simulink model "Gate_Splitter_x4"  (Simulink 6.6)
settings: Solver=ode45  StartTime=0.0  StopTime=5000/144e6  RelTol=1e-3
libraries: xbsIndex_r4 x205, simulink x1
(part 1 of 2)
settings Model: Creator=tbrimeye  LastModifiedBy=tbrimeye
settings DebuggingCC: SignalResolutionControl=TryResolveAllWithWarning  MultiTaskDSMMsg=warning  MultiTaskCondExecSysMsg=none
settings RTWCC: IncludeERTFirstTime=on

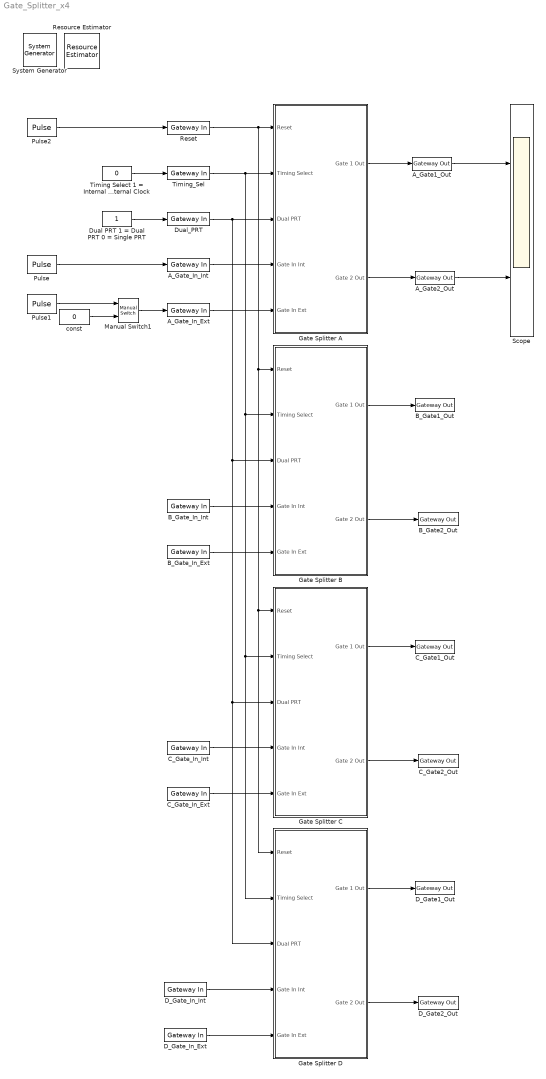
== system Gate_Splitter_x4 ==
  " System Generator" : xbsIndex_r4/ System Generator  Tag=genX  SystemSampleTime=-1  xilinxfamily=virtex4  part=xc4vsx35  speed=-11  package=ff668  synthesis_tool=XST  directory=C:/Work_Projects/Xilinx/SysGen_Outputs/Gate_Splitter  testbench=off  simulink_period=1/60e6  sysclk_period=(1/60e6)*1e9  incr_netlist=off  trim_vbits=Everywhere in SubSystem  dbl_ovrd=According to Block Masks  core_generation=According to Block Masks  run_coregen=off  deprecated_control=off  eval_field=0  block_type=sysgen
      settings: block_version=8.2
  A_Gate1_Out : xbsIndex_r4/Gateway Out  hdl_port=on  timing_constraint=None  locs_specified=off  LOCs={}  block_type=gatewayout
      settings: infoedit="Gateway out block.  Converts Xilinx fixed point inputs into ouputs of type Simulink integer, double, or fixed point.<P><P>Hardware notes:  In hardware these blocks become top level output ports or are discarded, depending on how they are configured."  xl_area=[0 0 0 0 18 0 0]  block_version=VER_STRING_GOES_HERE
  A_Gate2_Out : xbsIndex_r4/Gateway Out  hdl_port=on  timing_constraint=None  locs_specified=off  LOCs={}  block_type=gatewayout
      settings: infoedit="Gateway out block.  Converts Xilinx fixed point inputs into ouputs of type Simulink integer, double, or fixed point.<P><P>Hardware notes:  In hardware these blocks become top level output ports or are discarded, depending on how they are configured."  xl_area=[0 0 0 0 18 0 0]  block_version=VER_STRING_GOES_HERE
  A_Gate_In_Ext : xbsIndex_r4/Gateway In  arith_type=Boolean  n_bits=18  bin_pt=0  quantization="Round  (unbiased: +/- Inf)"  overflow=Flag as error  period=1/60e6  dbl_ovrd=off  timing_constraint=None  locs_specified=off  LOCs={}  block_type=gatewayin
      settings: infoedit="Gateway in block.  Converts inputs of type Simulink integer, double and fixed point to  Xilinx fixed point type.<P><P>Hardware notes:  In hardware these blocks become top level input ports."  xl_area=[0 0 0 0 1 0 0]  block_version=8.2
  A_Gate_In_Int : xbsIndex_r4/Gateway In  arith_type=Boolean  n_bits=1  bin_pt=0  quantization="Round  (unbiased: +/- Inf)"  overflow=Flag as error  period=1/60e6  dbl_ovrd=off  timing_constraint=None  locs_specified=off  LOCs={}  block_type=gatewayin
      settings: infoedit="Gateway in block.  Converts inputs of type Simulink integer, double and fixed point to  Xilinx fixed point type.<P><P>Hardware notes:  In hardware these blocks become top level input ports."  xl_area=[0 0 0 0 1 0 0]  block_version=8.2
  B_Gate1_Out : xbsIndex_r4/Gateway Out  hdl_port=on  timing_constraint=None  locs_specified=off  LOCs={}  block_type=gatewayout
      settings: infoedit="Gateway out block.  Converts Xilinx fixed point inputs into ouputs of type Simulink integer, double, or fixed point.<P><P>Hardware notes:  In hardware these blocks become top level output ports or are discarded, depending on how they are configured."  xl_area=[0 0 0 0 18 0 0]  block_version=VER_STRING_GOES_HERE
  B_Gate2_Out : xbsIndex_r4/Gateway Out  hdl_port=on  timing_constraint=None  locs_specified=off  LOCs={}  block_type=gatewayout
      settings: infoedit="Gateway out block.  Converts Xilinx fixed point inputs into ouputs of type Simulink integer, double, or fixed point.<P><P>Hardware notes:  In hardware these blocks become top level output ports or are discarded, depending on how they are configured."  xl_area=[0 0 0 0 18 0 0]  block_version=VER_STRING_GOES_HERE
  B_Gate_In_Ext : xbsIndex_r4/Gateway In  arith_type=Boolean  n_bits=18  bin_pt=0  quantization="Round  (unbiased: +/- Inf)"  overflow=Flag as error  period=1/60e6  dbl_ovrd=off  timing_constraint=None  locs_specified=off  LOCs={}  block_type=gatewayin
      settings: infoedit="Gateway in block.  Converts inputs of type Simulink integer, double and fixed point to  Xilinx fixed point type.<P><P>Hardware notes:  In hardware these blocks become top level input ports."  xl_area=[0 0 0 0 1 0 0]  block_version=8.2
  B_Gate_In_Int : xbsIndex_r4/Gateway In  arith_type=Boolean  n_bits=1  bin_pt=0  quantization="Round  (unbiased: +/- Inf)"  overflow=Flag as error  period=1/60e6  dbl_ovrd=off  timing_constraint=None  locs_specified=off  LOCs={}  block_type=gatewayin
      settings: infoedit="Gateway in block.  Converts inputs of type Simulink integer, double and fixed point to  Xilinx fixed point type.<P><P>Hardware notes:  In hardware these blocks become top level input ports."  xl_area=[0 0 0 0 1 0 0]  block_version=8.2
  C_Gate1_Out : xbsIndex_r4/Gateway Out  hdl_port=on  timing_constraint=None  locs_specified=off  LOCs={}  block_type=gatewayout
      settings: infoedit="Gateway out block.  Converts Xilinx fixed point inputs into ouputs of type Simulink integer, double, or fixed point.<P><P>Hardware notes:  In hardware these blocks become top level output ports or are discarded, depending on how they are configured."  xl_area=[0 0 0 0 18 0 0]  block_version=VER_STRING_GOES_HERE
  C_Gate2_Out : xbsIndex_r4/Gateway Out  hdl_port=on  timing_constraint=None  locs_specified=off  LOCs={}  block_type=gatewayout
      settings: infoedit="Gateway out block.  Converts Xilinx fixed point inputs into ouputs of type Simulink integer, double, or fixed point.<P><P>Hardware notes:  In hardware these blocks become top level output ports or are discarded, depending on how they are configured."  xl_area=[0 0 0 0 18 0 0]  block_version=VER_STRING_GOES_HERE
  C_Gate_In_Ext : xbsIndex_r4/Gateway In  arith_type=Boolean  n_bits=18  bin_pt=0  quantization="Round  (unbiased: +/- Inf)"  overflow=Flag as error  period=1/60e6  dbl_ovrd=off  timing_constraint=None  locs_specified=off  LOCs={}  block_type=gatewayin
      settings: infoedit="Gateway in block.  Converts inputs of type Simulink integer, double and fixed point to  Xilinx fixed point type.<P><P>Hardware notes:  In hardware these blocks become top level input ports."  xl_area=[0 0 0 0 1 0 0]  block_version=8.2
  C_Gate_In_Int : xbsIndex_r4/Gateway In  arith_type=Boolean  n_bits=1  bin_pt=0  quantization="Round  (unbiased: +/- Inf)"  overflow=Flag as error  period=1/60e6  dbl_ovrd=off  timing_constraint=None  locs_specified=off  LOCs={}  block_type=gatewayin
      settings: infoedit="Gateway in block.  Converts inputs of type Simulink integer, double and fixed point to  Xilinx fixed point type.<P><P>Hardware notes:  In hardware these blocks become top level input ports."  xl_area=[0 0 0 0 1 0 0]  block_version=8.2
  D_Gate1_Out : xbsIndex_r4/Gateway Out  hdl_port=on  timing_constraint=None  locs_specified=off  LOCs={}  block_type=gatewayout
      settings: infoedit="Gateway out block.  Converts Xilinx fixed point inputs into ouputs of type Simulink integer, double, or fixed point.<P><P>Hardware notes:  In hardware these blocks become top level output ports or are discarded, depending on how they are configured."  xl_area=[0 0 0 0 18 0 0]  block_version=VER_STRING_GOES_HERE
  D_Gate2_Out : xbsIndex_r4/Gateway Out  hdl_port=on  timing_constraint=None  locs_specified=off  LOCs={}  block_type=gatewayout
      settings: infoedit="Gateway out block.  Converts Xilinx fixed point inputs into ouputs of type Simulink integer, double, or fixed point.<P><P>Hardware notes:  In hardware these blocks become top level output ports or are discarded, depending on how they are configured."  xl_area=[0 0 0 0 18 0 0]  block_version=VER_STRING_GOES_HERE
  D_Gate_In_Ext : xbsIndex_r4/Gateway In  arith_type=Boolean  n_bits=18  bin_pt=0  quantization="Round  (unbiased: +/- Inf)"  overflow=Flag as error  period=1/60e6  dbl_ovrd=off  timing_constraint=None  locs_specified=off  LOCs={}  block_type=gatewayin
      settings: infoedit="Gateway in block.  Converts inputs of type Simulink integer, double and fixed point to  Xilinx fixed point type.<P><P>Hardware notes:  In hardware these blocks become top level input ports."  xl_area=[0 0 0 0 1 0 0]  block_version=8.2
  D_Gate_In_Int : xbsIndex_r4/Gateway In  arith_type=Boolean  n_bits=1  bin_pt=0  quantization="Round  (unbiased: +/- Inf)"  overflow=Flag as error  period=1/60e6  dbl_ovrd=off  timing_constraint=None  locs_specified=off  LOCs={}  block_type=gatewayin
      settings: infoedit="Gateway in block.  Converts inputs of type Simulink integer, double and fixed point to  Xilinx fixed point type.<P><P>Hardware notes:  In hardware these blocks become top level input ports."  xl_area=[0 0 0 0 1 0 0]  block_version=8.2
  Dual PRT 1 = Dual PRT 0 = Single PRT : Constant
  Dual_PRT : xbsIndex_r4/Gateway In  arith_type=Boolean  n_bits=1  bin_pt=0  quantization="Round  (unbiased: +/- Inf)"  overflow=Flag as error  period=1/60e6  dbl_ovrd=off  timing_constraint=None  locs_specified=off  LOCs={}  block_type=gatewayin
      settings: infoedit="Gateway in block.  Converts inputs of type Simulink integer, double and fixed point to  Xilinx fixed point type.<P><P>Hardware notes:  In hardware these blocks become top level input ports."  xl_area=[0 0 0 0 1 0 0]  block_version=8.2
  Gate Splitter A : Subsystem
  Gate Splitter B : Subsystem
  Gate Splitter C : Subsystem
  Gate Splitter D : Subsystem
  Manual Switch1 : simulink/Signal Routing/Manual Switch  SystemSampleTime=-1  sw=1  action=0  varsize=off
  Pulse : DiscretePulseGenerator  PulseType=Time based  Period=500/144e6  PulseWidth=50  PhaseDelay=100/144e6
  Pulse1 : DiscretePulseGenerator  PulseType=Time based  Period=500/144e6  PulseWidth=20  PhaseDelay=100/144e6
  Pulse2 : DiscretePulseGenerator  PulseType=Time based  Period=5000/144e6
  Reset : xbsIndex_r4/Gateway In  arith_type=Boolean  n_bits=1  bin_pt=0  quantization="Round  (unbiased: +/- Inf)"  overflow=Flag as error  period=1/60e6  dbl_ovrd=off  timing_constraint=None  locs_specified=off  LOCs={}  block_type=gatewayin
      settings: infoedit="Gateway in block.  Converts inputs of type Simulink integer, double and fixed point to  Xilinx fixed point type.<P><P>Hardware notes:  In hardware these blocks become top level input ports."  xl_area=[0 0 0 0 1 0 0]  block_version=8.2
  Resource Estimator : xbsIndex_r4/Resource Estimator  Tag=resEstTag  Slices=925  FFs=1405  BRAMs=7  LUTs=1104  IOBs=133  EBMs=14  TBUFs=0  xl_use_estimator_area=off  est_options=Post Map  xl_estimator_area=[1915 2342 0 3405 33 4 0]  block_type=resource_estimator
      settings: AttributesFormatString=Resource\nEstimator  block_version=8.2
  Scope : Scope  NumInputPorts=2
      settings: YMin=-5~-5  YMax=5~5
  Timing Select 1 = Internal Clock 0 = External Clock : Constant  Value=0
  Timing_Sel : xbsIndex_r4/Gateway In  arith_type=Boolean  n_bits=1  bin_pt=0  quantization="Round  (unbiased: +/- Inf)"  overflow=Flag as error  period=1/60e6  dbl_ovrd=off  timing_constraint=None  locs_specified=off  LOCs={}  block_type=gatewayin
      settings: infoedit="Gateway in block.  Converts inputs of type Simulink integer, double and fixed point to  Xilinx fixed point type.<P><P>Hardware notes:  In hardware these blocks become top level input ports."  xl_area=[0 0 0 0 1 0 0]  block_version=8.2
  const : Constant  Value=0
  wires:
  Pulse/1 -> A_Gate_In_Int/1
  Pulse1/1 -> Manual Switch1/1
  const/1 -> Manual Switch1/2
  Manual Switch1/1 -> A_Gate_In_Ext/1
  Dual PRT 1 = Dual PRT 0 = Single PRT/1 -> Dual_PRT/1
  Timing Select 1 = Internal Clock 0 = External Clock/1 -> Timing_Sel/1
  Pulse2/1 -> Reset/1
  Reset/1 -> Gate Splitter C/1(Reset), Gate Splitter D/1(Reset), Gate Splitter B/1(Reset), Gate Splitter A/1(Reset)
  Timing_Sel/1 -> Gate Splitter C/2(Timing Select), Gate Splitter D/2(Timing Select), Gate Splitter B/2(Timing Select), Gate Splitter A/2(Timing Select)
  Dual_PRT/1 -> Gate Splitter C/3(Dual PRT), Gate Splitter D/3(Dual PRT), Gate Splitter B/3(Dual PRT), Gate Splitter A/3(Dual PRT)
  A_Gate_In_Int/1 -> Gate Splitter A/4(Gate In Int)
  A_Gate_In_Ext/1 -> Gate Splitter A/5(Gate In Ext)
  Gate Splitter A/1(Gate 1 Out) -> A_Gate1_Out/1
  Gate Splitter A/2(Gate 2 Out) -> A_Gate2_Out/1
  B_Gate_In_Int/1 -> Gate Splitter B/4(Gate In Int)
  B_Gate_In_Ext/1 -> Gate Splitter B/5(Gate In Ext)
  C_Gate_In_Int/1 -> Gate Splitter C/4(Gate In Int)
  C_Gate_In_Ext/1 -> Gate Splitter C/5(Gate In Ext)
  D_Gate_In_Int/1 -> Gate Splitter D/4(Gate In Int)
  D_Gate_In_Ext/1 -> Gate Splitter D/5(Gate In Ext)
  Gate Splitter B/1(Gate 1 Out) -> B_Gate1_Out/1
  Gate Splitter B/2(Gate 2 Out) -> B_Gate2_Out/1
  Gate Splitter C/1(Gate 1 Out) -> C_Gate1_Out/1
  Gate Splitter C/2(Gate 2 Out) -> C_Gate2_Out/1
  Gate Splitter D/1(Gate 1 Out) -> D_Gate1_Out/1
  Gate Splitter D/2(Gate 2 Out) -> D_Gate2_Out/1
  A_Gate1_Out/1 -> Scope/1
  A_Gate2_Out/1 -> Scope/2

== system Gate_Splitter_x4/Gate Splitter A ==
  Reset : Inport
  Timing Select : Inport  Port=2
  Dual PRT : Inport  Port=3
  Gate In Int : Inport  Port=4
  Gate In Ext : Inport  Port=5
  Gate Splitter : Subsystem
  Noise Cancellation : Subsystem
  Noise Cancellation1 : Subsystem
  Gate 1 Out : Outport
  Gate 2 Out : Outport  Port=2
  wires:
  Noise Cancellation/1(Gate Out) -> Gate Splitter/4(Gate In Int)
  Noise Cancellation1/1(Gate Out) -> Gate Splitter/5(Gate In Ext)
  Reset/1 -> Gate Splitter/1(Reset)
  Gate In Int/1 -> Noise Cancellation/1(Gate In)
  Gate In Ext/1 -> Noise Cancellation1/1(Gate In)
  Gate Splitter/1(Gate 1 Out) -> Gate 1 Out/1
  Timing Select/1 -> Gate Splitter/2(Timing Sel)
  Dual PRT/1 -> Gate Splitter/3(Dual PRT)
  Gate Splitter/2(Gate 2 Out) -> Gate 2 Out/1

== system Gate_Splitter_x4/Gate Splitter B ==
  Reset : Inport
  Timing Select : Inport  Port=2
  Dual PRT : Inport  Port=3
  Gate In Int : Inport  Port=4
  Gate In Ext : Inport  Port=5
  Gate Splitter : Subsystem
  Noise Cancellation : Subsystem
  Noise Cancellation1 : Subsystem
  Gate 1 Out : Outport
  Gate 2 Out : Outport  Port=2
  wires:
  Noise Cancellation/1(Gate Out) -> Gate Splitter/4(Gate In Int)
  Noise Cancellation1/1(Gate Out) -> Gate Splitter/5(Gate In Ext)
  Reset/1 -> Gate Splitter/1(Reset)
  Gate In Int/1 -> Noise Cancellation/1(Gate In)
  Gate In Ext/1 -> Noise Cancellation1/1(Gate In)
  Gate Splitter/1(Gate 1 Out) -> Gate 1 Out/1
  Timing Select/1 -> Gate Splitter/2(Timing Sel)
  Dual PRT/1 -> Gate Splitter/3(Dual PRT)
  Gate Splitter/2(Gate 2 Out) -> Gate 2 Out/1

== system Gate_Splitter_x4/Gate Splitter C ==
  Reset : Inport
  Timing Select : Inport  Port=2
  Dual PRT : Inport  Port=3
  Gate In Int : Inport  Port=4
  Gate In Ext : Inport  Port=5
  Gate Splitter : Subsystem
  Noise Cancellation : Subsystem
  Noise Cancellation1 : Subsystem
  Gate 1 Out : Outport
  Gate 2 Out : Outport  Port=2
  wires:
  Noise Cancellation/1(Gate Out) -> Gate Splitter/4(Gate In Int)
  Noise Cancellation1/1(Gate Out) -> Gate Splitter/5(Gate In Ext)
  Reset/1 -> Gate Splitter/1(Reset)
  Gate In Int/1 -> Noise Cancellation/1(Gate In)
  Gate In Ext/1 -> Noise Cancellation1/1(Gate In)
  Gate Splitter/1(Gate 1 Out) -> Gate 1 Out/1
  Timing Select/1 -> Gate Splitter/2(Timing Sel)
  Dual PRT/1 -> Gate Splitter/3(Dual PRT)
  Gate Splitter/2(Gate 2 Out) -> Gate 2 Out/1

== system Gate_Splitter_x4/Gate Splitter D ==
  Reset : Inport
  Timing Select : Inport  Port=2
  Dual PRT : Inport  Port=3
  Gate In Int : Inport  Port=4
  Gate In Ext : Inport  Port=5
  Gate Splitter : Subsystem
  Noise Cancellation : Subsystem
  Noise Cancellation1 : Subsystem
  Gate 1 Out : Outport
  Gate 2 Out : Outport  Port=2
  wires:
  Noise Cancellation/1(Gate Out) -> Gate Splitter/4(Gate In Int)
  Noise Cancellation1/1(Gate Out) -> Gate Splitter/5(Gate In Ext)
  Reset/1 -> Gate Splitter/1(Reset)
  Gate In Int/1 -> Noise Cancellation/1(Gate In)
  Gate In Ext/1 -> Noise Cancellation1/1(Gate In)
  Gate Splitter/1(Gate 1 Out) -> Gate 1 Out/1
  Timing Select/1 -> Gate Splitter/2(Timing Sel)
  Dual PRT/1 -> Gate Splitter/3(Dual PRT)
  Gate Splitter/2(Gate 2 Out) -> Gate 2 Out/1

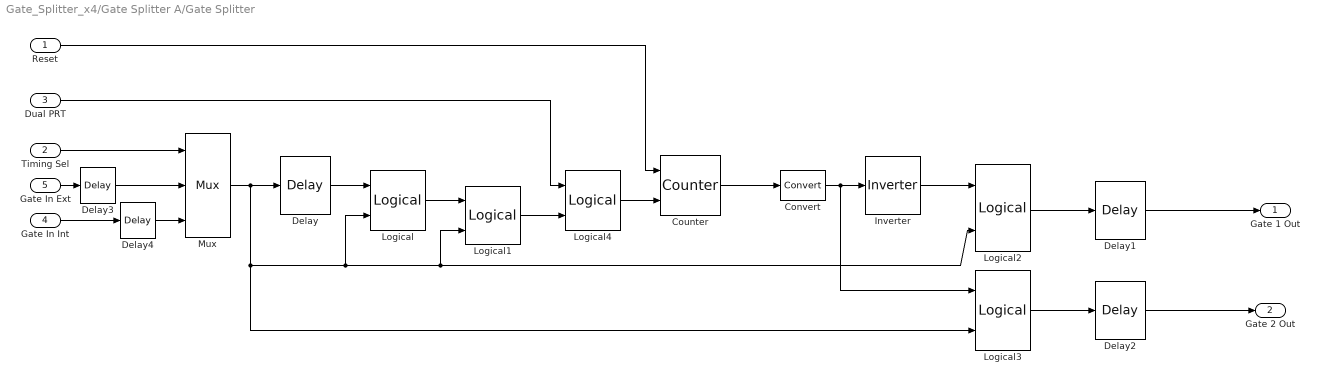
== system Gate_Splitter_x4/Gate Splitter A/Gate Splitter ==
  Reset : Inport
  Timing Sel : Inport  Port=2
  Dual PRT : Inport  Port=3
  Gate In Int : Inport  Port=4
  Gate In Ext : Inport  Port=5
  Convert : xbsIndex_r4/Convert  arith_type=Boolean  n_bits=16  bin_pt=14  quantization=Truncate  overflow=Wrap  latency=0  dbl_ovrd=off  pipeline=off  block_type=convert
      settings: block_version=8.2
  Counter : xbsIndex_r4/Counter  cnt_type=Free Running  cnt_to=Inf  operation=Up  start_count=0  cnt_by_val=1  arith_type=Unsigned  n_bits=1  bin_pt=0  load_pin=off  rst=on  en=on  explicit_period=on  period=1/60e6  dbl_ovrd=off  use_behavioral_HDL=off  use_rpm=off  block_type=counter
      settings: block_version=8.2
  Delay : xbsIndex_r4/Delay  en=off  latency=1  dbl_ovrd=off  reg_retiming=off  block_type=delay
      settings: infoedit=Hardware notes: A delay line is a chain, each link of which is an SRL16 followed by a flip-flop. If register retiming is enabled, the delay line is a chain of flip-flops.  block_version=8.2
  Delay1 : xbsIndex_r4/Delay  en=off  latency=279  dbl_ovrd=off  reg_retiming=off  block_type=delay
      settings: infoedit=Hardware notes: A delay line is a chain, each link of which is an SRL16 followed by a flip-flop. If register retiming is enabled, the delay line is a chain of flip-flops.  block_version=8.2
  Delay2 : xbsIndex_r4/Delay  en=off  latency=279  dbl_ovrd=off  reg_retiming=off  block_type=delay
      settings: infoedit=Hardware notes: A delay line is a chain, each link of which is an SRL16 followed by a flip-flop. If register retiming is enabled, the delay line is a chain of flip-flops.  block_version=8.2
  Delay3 : xbsIndex_r4/Delay  en=off  latency=1  dbl_ovrd=off  reg_retiming=off  block_type=delay
      settings: infoedit=Hardware notes: A delay line is a chain, each link of which is an SRL16 followed by a flip-flop. If register retiming is enabled, the delay line is a chain of flip-flops.  block_version=8.2
  Delay4 : xbsIndex_r4/Delay  en=off  latency=1  dbl_ovrd=off  reg_retiming=off  block_type=delay
      settings: infoedit=Hardware notes: A delay line is a chain, each link of which is an SRL16 followed by a flip-flop. If register retiming is enabled, the delay line is a chain of flip-flops.  block_version=8.2
  Inverter : xbsIndex_r4/Inverter  en=off  latency=0  dbl_ovrd=off  block_type=inv
      settings: block_version=8.2
  Logical : xbsIndex_r4/Logical  logical_function=OR  inputs=2  en=off  latency=0  precision=Full  arith_type=Unsigned  n_bits=16  bin_pt=0  align_bp=on  dbl_ovrd=off  block_type=logical
      settings: block_version=8.2
  Logical1 : xbsIndex_r4/Logical  logical_function=XOR  inputs=2  en=off  latency=0  precision=Full  arith_type=Unsigned  n_bits=16  bin_pt=0  align_bp=on  dbl_ovrd=off  block_type=logical
      settings: block_version=8.2
  Logical2 : xbsIndex_r4/Logical  logical_function=AND  inputs=2  en=off  latency=0  precision=Full  arith_type=Unsigned  n_bits=16  bin_pt=0  align_bp=on  dbl_ovrd=off  block_type=logical
      settings: block_version=8.2
  Logical3 : xbsIndex_r4/Logical  logical_function=AND  inputs=2  en=off  latency=0  precision=Full  arith_type=Unsigned  n_bits=16  bin_pt=0  align_bp=on  dbl_ovrd=off  block_type=logical
      settings: block_version=8.2
  Logical4 : xbsIndex_r4/Logical  logical_function=AND  inputs=2  en=off  latency=0  precision=Full  arith_type=Unsigned  n_bits=16  bin_pt=0  align_bp=on  dbl_ovrd=off  block_type=logical
      settings: block_version=8.2
  Mux : xbsIndex_r4/Mux  inputs=2  en=off  latency=0  precision=Full  arith_type=Unsigned  n_bits=16  bin_pt=14  quantization=Truncate  overflow=Wrap  dbl_ovrd=off  block_type=mux
      settings: block_version=8.2
  Gate 1 Out : Outport
  Gate 2 Out : Outport  Port=2
  wires:
  Timing Sel/1 -> Mux/1
  Gate In Ext/1 -> Delay3/1
  Gate In Int/1 -> Delay4/1
  Mux/1 -> Delay/1, Logical/2, Logical2/2, Logical1/2, Logical3/2
  Delay/1 -> Logical/1
  Logical/1 -> Logical1/1
  Counter/1 -> Convert/1
  Inverter/1 -> Logical2/1
  Logical3/1 -> Delay2/1
  Logical2/1 -> Delay1/1
  Convert/1 -> Inverter/1, Logical3/1
  Logical1/1 -> Logical4/2
  Dual PRT/1 -> Logical4/1
  Logical4/1 -> Counter/2
  Reset/1 -> Counter/1
  Delay1/1 -> Gate 1 Out/1
  Delay2/1 -> Gate 2 Out/1
  Delay3/1 -> Mux/2
  Delay4/1 -> Mux/3

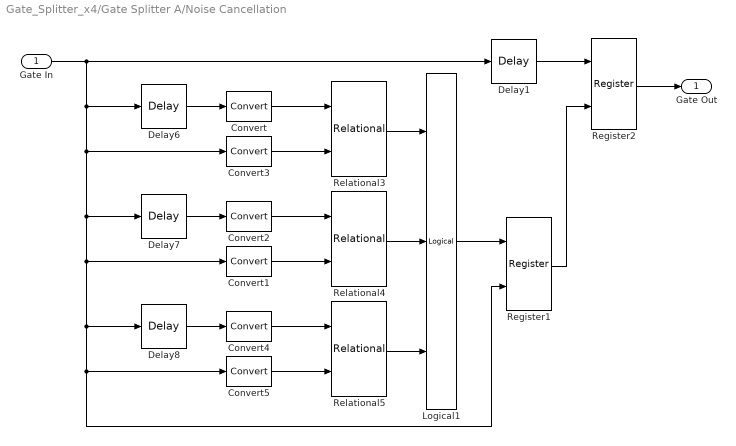
== system Gate_Splitter_x4/Gate Splitter A/Noise Cancellation ==
  Gate In : Inport
  Convert{,1..5} (6 alike) : xbsIndex_r4/Convert  arith_type=Unsigned  n_bits=1  bin_pt=0  quantization=Truncate  overflow=Saturate  latency=0  dbl_ovrd=off  pipeline=off  block_type=convert
      settings: block_version=8.2
  Delay1 : xbsIndex_r4/Delay  en=off  latency=4  dbl_ovrd=off  reg_retiming=off  block_type=delay
      settings: infoedit=Hardware notes: A delay line is a chain, each link of which is an SRL16 followed by a flip-flop. If register retiming is enabled, the delay line is a chain of flip-flops.  block_version=8.2
  Delay6 : xbsIndex_r4/Delay  en=off  latency=1  dbl_ovrd=off  reg_retiming=off  block_type=delay
      settings: infoedit=Hardware notes: A delay line is a chain, each link of which is an SRL16 followed by a flip-flop. If register retiming is enabled, the delay line is a chain of flip-flops.  block_version=8.2
  Delay7 : xbsIndex_r4/Delay  en=off  latency=2  dbl_ovrd=off  reg_retiming=off  block_type=delay
      settings: infoedit=Hardware notes: A delay line is a chain, each link of which is an SRL16 followed by a flip-flop. If register retiming is enabled, the delay line is a chain of flip-flops.  block_version=8.2
  Delay8 : xbsIndex_r4/Delay  en=off  latency=3  dbl_ovrd=off  reg_retiming=off  block_type=delay
      settings: infoedit=Hardware notes: A delay line is a chain, each link of which is an SRL16 followed by a flip-flop. If register retiming is enabled, the delay line is a chain of flip-flops.  block_version=8.2
  Logical1 : xbsIndex_r4/Logical  logical_function=OR  inputs=3  en=off  latency=0  precision=Full  arith_type=Unsigned  n_bits=16  bin_pt=0  align_bp=on  dbl_ovrd=off  block_type=logical
      settings: block_version=8.2
  Register1 : xbsIndex_r4/Register  init=0  rst=off  en=on  dbl_ovrd=off  block_type=register
      settings: block_version=8.2
  Register2 : xbsIndex_r4/Register  init=0  rst=on  en=off  dbl_ovrd=off  block_type=register
      settings: block_version=8.2
  Relational3 : xbsIndex_r4/Relational  mode=a!=b  en=off  latency=2  dbl_ovrd=off  block_type=relational
      settings: block_version=8.2
  Relational4 : xbsIndex_r4/Relational  mode=a!=b  en=off  latency=1  dbl_ovrd=off  block_type=relational
      settings: block_version=8.2
  Relational5 : xbsIndex_r4/Relational  mode=a!=b  en=off  latency=0  dbl_ovrd=off  block_type=relational
      settings: block_version=8.2
  Gate Out : Outport
  wires:
  Convert/1 -> Relational3/1
  Delay6/1 -> Convert/1
  Convert2/1 -> Relational4/1
  Delay7/1 -> Convert2/1
  Convert4/1 -> Relational5/1
  Delay8/1 -> Convert4/1
  Convert5/1 -> Relational5/2
  Relational3/1 -> Logical1/1
  Relational4/1 -> Logical1/2
  Relational5/1 -> Logical1/3
  Convert3/1 -> Relational3/2
  Convert1/1 -> Relational4/2
  Delay1/1 -> Register2/1
  Logical1/1 -> Register1/1
  Register1/1 -> Register2/2
  Gate In/1 -> Delay6/1, Delay7/1, Delay8/1, Convert5/1, Register1/2, Convert1/1, Convert3/1, Delay1/1
  Register2/1 -> Gate Out/1

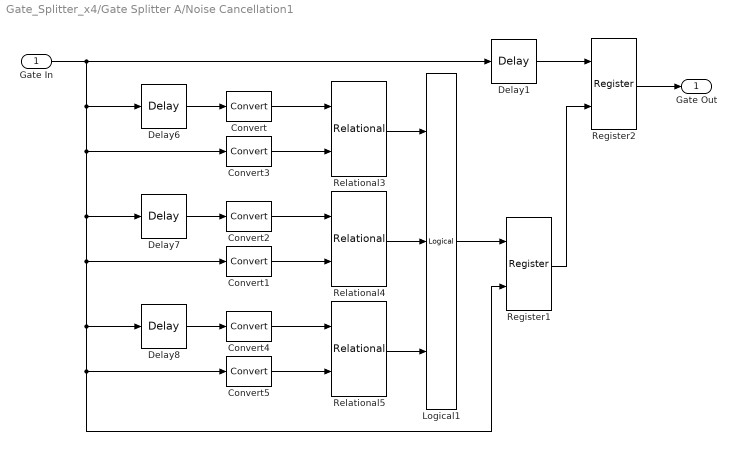
== system Gate_Splitter_x4/Gate Splitter A/Noise Cancellation1 ==
  Gate In : Inport
  Convert{,1..5} (6 alike) : xbsIndex_r4/Convert  arith_type=Unsigned  n_bits=1  bin_pt=0  quantization=Truncate  overflow=Saturate  latency=0  dbl_ovrd=off  pipeline=off  block_type=convert
      settings: block_version=8.2
  Delay1 : xbsIndex_r4/Delay  en=off  latency=4  dbl_ovrd=off  reg_retiming=off  block_type=delay
      settings: infoedit=Hardware notes: A delay line is a chain, each link of which is an SRL16 followed by a flip-flop. If register retiming is enabled, the delay line is a chain of flip-flops.  block_version=8.2
  Delay6 : xbsIndex_r4/Delay  en=off  latency=1  dbl_ovrd=off  reg_retiming=off  block_type=delay
      settings: infoedit=Hardware notes: A delay line is a chain, each link of which is an SRL16 followed by a flip-flop. If register retiming is enabled, the delay line is a chain of flip-flops.  block_version=8.2
  Delay7 : xbsIndex_r4/Delay  en=off  latency=2  dbl_ovrd=off  reg_retiming=off  block_type=delay
      settings: infoedit=Hardware notes: A delay line is a chain, each link of which is an SRL16 followed by a flip-flop. If register retiming is enabled, the delay line is a chain of flip-flops.  block_version=8.2
  Delay8 : xbsIndex_r4/Delay  en=off  latency=3  dbl_ovrd=off  reg_retiming=off  block_type=delay
      settings: infoedit=Hardware notes: A delay line is a chain, each link of which is an SRL16 followed by a flip-flop. If register retiming is enabled, the delay line is a chain of flip-flops.  block_version=8.2
  Logical1 : xbsIndex_r4/Logical  logical_function=OR  inputs=3  en=off  latency=0  precision=Full  arith_type=Unsigned  n_bits=16  bin_pt=0  align_bp=on  dbl_ovrd=off  block_type=logical
      settings: block_version=8.2
  Register1 : xbsIndex_r4/Register  init=0  rst=off  en=on  dbl_ovrd=off  block_type=register
      settings: block_version=8.2
  Register2 : xbsIndex_r4/Register  init=0  rst=on  en=off  dbl_ovrd=off  block_type=register
      settings: block_version=8.2
  Relational3 : xbsIndex_r4/Relational  mode=a!=b  en=off  latency=2  dbl_ovrd=off  block_type=relational
      settings: block_version=8.2
  Relational4 : xbsIndex_r4/Relational  mode=a!=b  en=off  latency=1  dbl_ovrd=off  block_type=relational
      settings: block_version=8.2
  Relational5 : xbsIndex_r4/Relational  mode=a!=b  en=off  latency=0  dbl_ovrd=off  block_type=relational
      settings: block_version=8.2
  Gate Out : Outport
  wires:
  Convert/1 -> Relational3/1
  Delay6/1 -> Convert/1
  Convert2/1 -> Relational4/1
  Delay7/1 -> Convert2/1
  Convert4/1 -> Relational5/1
  Delay8/1 -> Convert4/1
  Convert5/1 -> Relational5/2
  Relational3/1 -> Logical1/1
  Relational4/1 -> Logical1/2
  Relational5/1 -> Logical1/3
  Convert3/1 -> Relational3/2
  Convert1/1 -> Relational4/2
  Delay1/1 -> Register2/1
  Logical1/1 -> Register1/1
  Register1/1 -> Register2/2
  Gate In/1 -> Delay6/1, Delay7/1, Delay8/1, Convert5/1, Register1/2, Convert1/1, Convert3/1, Delay1/1
  Register2/1 -> Gate Out/1

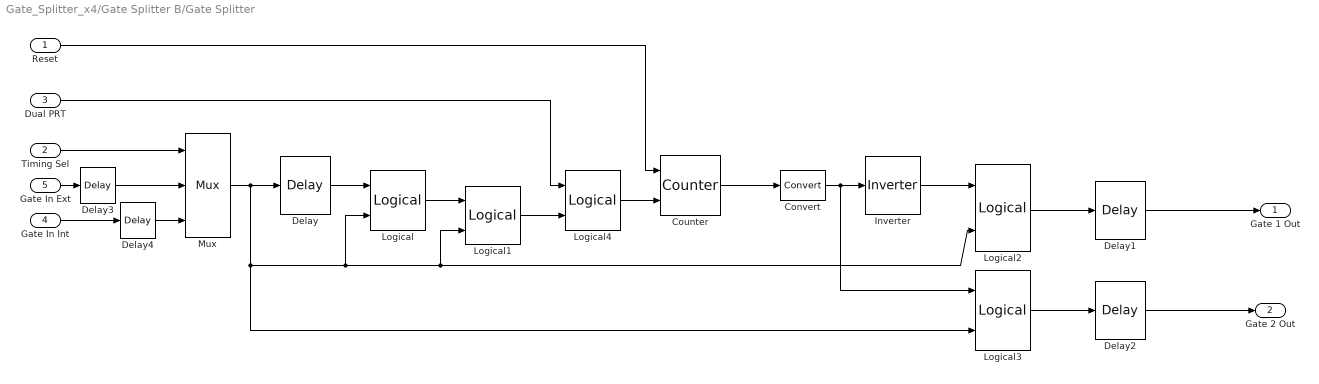
== system Gate_Splitter_x4/Gate Splitter B/Gate Splitter ==
  Reset : Inport
  Timing Sel : Inport  Port=2
  Dual PRT : Inport  Port=3
  Gate In Int : Inport  Port=4
  Gate In Ext : Inport  Port=5
  Convert : xbsIndex_r4/Convert  arith_type=Boolean  n_bits=16  bin_pt=14  quantization=Truncate  overflow=Wrap  latency=0  dbl_ovrd=off  pipeline=off  block_type=convert
      settings: block_version=8.2
  Counter : xbsIndex_r4/Counter  cnt_type=Free Running  cnt_to=Inf  operation=Up  start_count=0  cnt_by_val=1  arith_type=Unsigned  n_bits=1  bin_pt=0  load_pin=off  rst=on  en=on  explicit_period=on  period=1/60e6  dbl_ovrd=off  use_behavioral_HDL=off  use_rpm=off  block_type=counter
      settings: block_version=8.2
  Delay : xbsIndex_r4/Delay  en=off  latency=1  dbl_ovrd=off  reg_retiming=off  block_type=delay
      settings: infoedit=Hardware notes: A delay line is a chain, each link of which is an SRL16 followed by a flip-flop. If register retiming is enabled, the delay line is a chain of flip-flops.  block_version=8.2
  Delay1 : xbsIndex_r4/Delay  en=off  latency=279  dbl_ovrd=off  reg_retiming=off  block_type=delay
      settings: infoedit=Hardware notes: A delay line is a chain, each link of which is an SRL16 followed by a flip-flop. If register retiming is enabled, the delay line is a chain of flip-flops.  block_version=8.2
  Delay2 : xbsIndex_r4/Delay  en=off  latency=279  dbl_ovrd=off  reg_retiming=off  block_type=delay
      settings: infoedit=Hardware notes: A delay line is a chain, each link of which is an SRL16 followed by a flip-flop. If register retiming is enabled, the delay line is a chain of flip-flops.  block_version=8.2
  Delay3 : xbsIndex_r4/Delay  en=off  latency=1  dbl_ovrd=off  reg_retiming=off  block_type=delay
      settings: infoedit=Hardware notes: A delay line is a chain, each link of which is an SRL16 followed by a flip-flop. If register retiming is enabled, the delay line is a chain of flip-flops.  block_version=8.2
  Delay4 : xbsIndex_r4/Delay  en=off  latency=1  dbl_ovrd=off  reg_retiming=off  block_type=delay
      settings: infoedit=Hardware notes: A delay line is a chain, each link of which is an SRL16 followed by a flip-flop. If register retiming is enabled, the delay line is a chain of flip-flops.  block_version=8.2
  Inverter : xbsIndex_r4/Inverter  en=off  latency=0  dbl_ovrd=off  block_type=inv
      settings: block_version=8.2
  Logical : xbsIndex_r4/Logical  logical_function=OR  inputs=2  en=off  latency=0  precision=Full  arith_type=Unsigned  n_bits=16  bin_pt=0  align_bp=on  dbl_ovrd=off  block_type=logical
      settings: block_version=8.2
  Logical1 : xbsIndex_r4/Logical  logical_function=XOR  inputs=2  en=off  latency=0  precision=Full  arith_type=Unsigned  n_bits=16  bin_pt=0  align_bp=on  dbl_ovrd=off  block_type=logical
      settings: block_version=8.2
  Logical2 : xbsIndex_r4/Logical  logical_function=AND  inputs=2  en=off  latency=0  precision=Full  arith_type=Unsigned  n_bits=16  bin_pt=0  align_bp=on  dbl_ovrd=off  block_type=logical
      settings: block_version=8.2
  Logical3 : xbsIndex_r4/Logical  logical_function=AND  inputs=2  en=off  latency=0  precision=Full  arith_type=Unsigned  n_bits=16  bin_pt=0  align_bp=on  dbl_ovrd=off  block_type=logical
      settings: block_version=8.2
  Logical4 : xbsIndex_r4/Logical  logical_function=AND  inputs=2  en=off  latency=0  precision=Full  arith_type=Unsigned  n_bits=16  bin_pt=0  align_bp=on  dbl_ovrd=off  block_type=logical
      settings: block_version=8.2
  Mux : xbsIndex_r4/Mux  inputs=2  en=off  latency=0  precision=Full  arith_type=Unsigned  n_bits=16  bin_pt=14  quantization=Truncate  overflow=Wrap  dbl_ovrd=off  block_type=mux
      settings: block_version=8.2
  Gate 1 Out : Outport
  Gate 2 Out : Outport  Port=2
  wires:
  Timing Sel/1 -> Mux/1
  Gate In Ext/1 -> Delay3/1
  Gate In Int/1 -> Delay4/1
  Mux/1 -> Delay/1, Logical/2, Logical2/2, Logical1/2, Logical3/2
  Delay/1 -> Logical/1
  Logical/1 -> Logical1/1
  Counter/1 -> Convert/1
  Inverter/1 -> Logical2/1
  Logical3/1 -> Delay2/1
  Logical2/1 -> Delay1/1
  Convert/1 -> Inverter/1, Logical3/1
  Logical1/1 -> Logical4/2
  Dual PRT/1 -> Logical4/1
  Logical4/1 -> Counter/2
  Reset/1 -> Counter/1
  Delay1/1 -> Gate 1 Out/1
  Delay2/1 -> Gate 2 Out/1
  Delay3/1 -> Mux/2
  Delay4/1 -> Mux/3

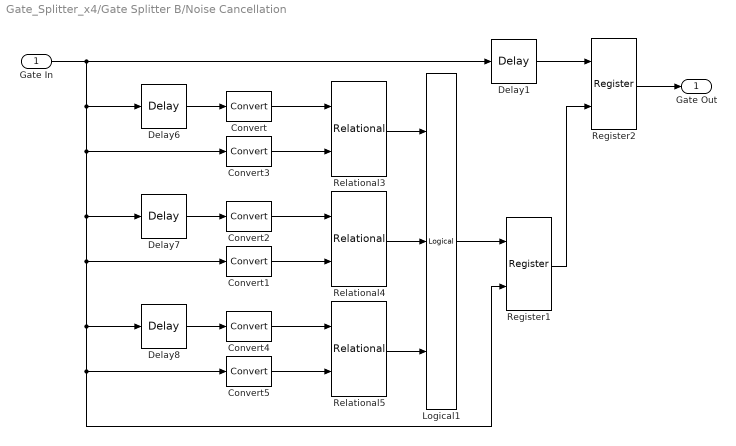
== system Gate_Splitter_x4/Gate Splitter B/Noise Cancellation ==
  Gate In : Inport
  Convert{,1..5} (6 alike) : xbsIndex_r4/Convert  arith_type=Unsigned  n_bits=1  bin_pt=0  quantization=Truncate  overflow=Saturate  latency=0  dbl_ovrd=off  pipeline=off  block_type=convert
      settings: block_version=8.2
  Delay1 : xbsIndex_r4/Delay  en=off  latency=4  dbl_ovrd=off  reg_retiming=off  block_type=delay
      settings: infoedit=Hardware notes: A delay line is a chain, each link of which is an SRL16 followed by a flip-flop. If register retiming is enabled, the delay line is a chain of flip-flops.  block_version=8.2
  Delay6 : xbsIndex_r4/Delay  en=off  latency=1  dbl_ovrd=off  reg_retiming=off  block_type=delay
      settings: infoedit=Hardware notes: A delay line is a chain, each link of which is an SRL16 followed by a flip-flop. If register retiming is enabled, the delay line is a chain of flip-flops.  block_version=8.2
  Delay7 : xbsIndex_r4/Delay  en=off  latency=2  dbl_ovrd=off  reg_retiming=off  block_type=delay
      settings: infoedit=Hardware notes: A delay line is a chain, each link of which is an SRL16 followed by a flip-flop. If register retiming is enabled, the delay line is a chain of flip-flops.  block_version=8.2
  Delay8 : xbsIndex_r4/Delay  en=off  latency=3  dbl_ovrd=off  reg_retiming=off  block_type=delay
      settings: infoedit=Hardware notes: A delay line is a chain, each link of which is an SRL16 followed by a flip-flop. If register retiming is enabled, the delay line is a chain of flip-flops.  block_version=8.2
  Logical1 : xbsIndex_r4/Logical  logical_function=OR  inputs=3  en=off  latency=0  precision=Full  arith_type=Unsigned  n_bits=16  bin_pt=0  align_bp=on  dbl_ovrd=off  block_type=logical
      settings: block_version=8.2
  Register1 : xbsIndex_r4/Register  init=0  rst=off  en=on  dbl_ovrd=off  block_type=register
      settings: block_version=8.2
  Register2 : xbsIndex_r4/Register  init=0  rst=on  en=off  dbl_ovrd=off  block_type=register
      settings: block_version=8.2
  Relational3 : xbsIndex_r4/Relational  mode=a!=b  en=off  latency=2  dbl_ovrd=off  block_type=relational
      settings: block_version=8.2
  Relational4 : xbsIndex_r4/Relational  mode=a!=b  en=off  latency=1  dbl_ovrd=off  block_type=relational
      settings: block_version=8.2
  Relational5 : xbsIndex_r4/Relational  mode=a!=b  en=off  latency=0  dbl_ovrd=off  block_type=relational
      settings: block_version=8.2
  Gate Out : Outport
  wires:
  Convert/1 -> Relational3/1
  Delay6/1 -> Convert/1
  Convert2/1 -> Relational4/1
  Delay7/1 -> Convert2/1
  Convert4/1 -> Relational5/1
  Delay8/1 -> Convert4/1
  Convert5/1 -> Relational5/2
  Relational3/1 -> Logical1/1
  Relational4/1 -> Logical1/2
  Relational5/1 -> Logical1/3
  Convert3/1 -> Relational3/2
  Convert1/1 -> Relational4/2
  Delay1/1 -> Register2/1
  Logical1/1 -> Register1/1
  Register1/1 -> Register2/2
  Gate In/1 -> Delay6/1, Delay7/1, Delay8/1, Convert5/1, Register1/2, Convert1/1, Convert3/1, Delay1/1
  Register2/1 -> Gate Out/1

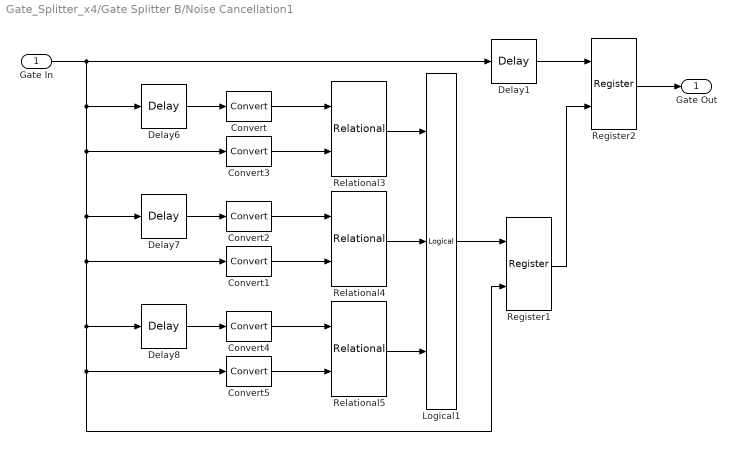
== system Gate_Splitter_x4/Gate Splitter B/Noise Cancellation1 ==
  Gate In : Inport
  Convert{,1..5} (6 alike) : xbsIndex_r4/Convert  arith_type=Unsigned  n_bits=1  bin_pt=0  quantization=Truncate  overflow=Saturate  latency=0  dbl_ovrd=off  pipeline=off  block_type=convert
      settings: block_version=8.2
  Delay1 : xbsIndex_r4/Delay  en=off  latency=4  dbl_ovrd=off  reg_retiming=off  block_type=delay
      settings: infoedit=Hardware notes: A delay line is a chain, each link of which is an SRL16 followed by a flip-flop. If register retiming is enabled, the delay line is a chain of flip-flops.  block_version=8.2
  Delay6 : xbsIndex_r4/Delay  en=off  latency=1  dbl_ovrd=off  reg_retiming=off  block_type=delay
      settings: infoedit=Hardware notes: A delay line is a chain, each link of which is an SRL16 followed by a flip-flop. If register retiming is enabled, the delay line is a chain of flip-flops.  block_version=8.2
  Delay7 : xbsIndex_r4/Delay  en=off  latency=2  dbl_ovrd=off  reg_retiming=off  block_type=delay
      settings: infoedit=Hardware notes: A delay line is a chain, each link of which is an SRL16 followed by a flip-flop. If register retiming is enabled, the delay line is a chain of flip-flops.  block_version=8.2
  Delay8 : xbsIndex_r4/Delay  en=off  latency=3  dbl_ovrd=off  reg_retiming=off  block_type=delay
      settings: infoedit=Hardware notes: A delay line is a chain, each link of which is an SRL16 followed by a flip-flop. If register retiming is enabled, the delay line is a chain of flip-flops.  block_version=8.2
  Logical1 : xbsIndex_r4/Logical  logical_function=OR  inputs=3  en=off  latency=0  precision=Full  arith_type=Unsigned  n_bits=16  bin_pt=0  align_bp=on  dbl_ovrd=off  block_type=logical
      settings: block_version=8.2
  Register1 : xbsIndex_r4/Register  init=0  rst=off  en=on  dbl_ovrd=off  block_type=register
      settings: block_version=8.2
  Register2 : xbsIndex_r4/Register  init=0  rst=on  en=off  dbl_ovrd=off  block_type=register
      settings: block_version=8.2
  Relational3 : xbsIndex_r4/Relational  mode=a!=b  en=off  latency=2  dbl_ovrd=off  block_type=relational
      settings: block_version=8.2
  Relational4 : xbsIndex_r4/Relational  mode=a!=b  en=off  latency=1  dbl_ovrd=off  block_type=relational
      settings: block_version=8.2
  Relational5 : xbsIndex_r4/Relational  mode=a!=b  en=off  latency=0  dbl_ovrd=off  block_type=relational
      settings: block_version=8.2
  Gate Out : Outport
  wires:
  Convert/1 -> Relational3/1
  Delay6/1 -> Convert/1
  Convert2/1 -> Relational4/1
  Delay7/1 -> Convert2/1
  Convert4/1 -> Relational5/1
  Delay8/1 -> Convert4/1
  Convert5/1 -> Relational5/2
  Relational3/1 -> Logical1/1
  Relational4/1 -> Logical1/2
  Relational5/1 -> Logical1/3
  Convert3/1 -> Relational3/2
  Convert1/1 -> Relational4/2
  Delay1/1 -> Register2/1
  Logical1/1 -> Register1/1
  Register1/1 -> Register2/2
  Gate In/1 -> Delay6/1, Delay7/1, Delay8/1, Convert5/1, Register1/2, Convert1/1, Convert3/1, Delay1/1
  Register2/1 -> Gate Out/1

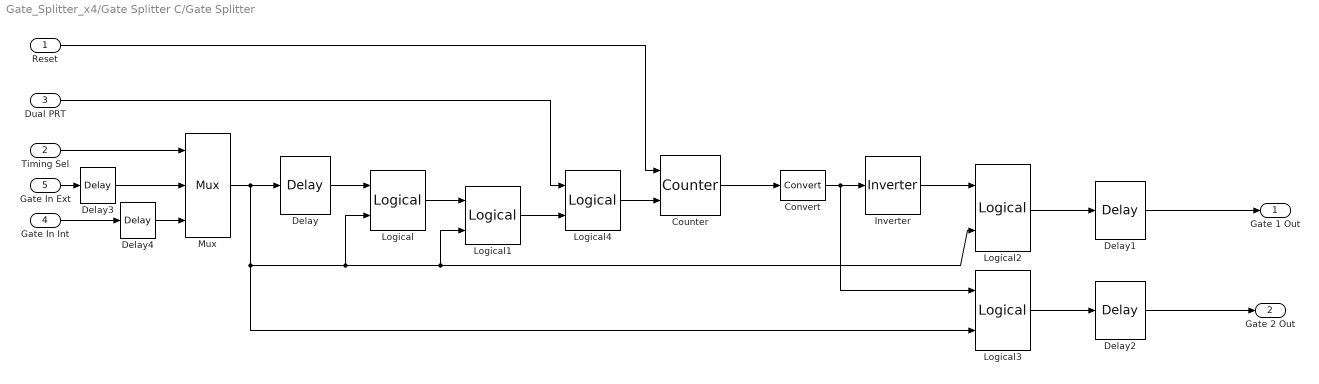
== system Gate_Splitter_x4/Gate Splitter C/Gate Splitter ==
  Reset : Inport
  Timing Sel : Inport  Port=2
  Dual PRT : Inport  Port=3
  Gate In Int : Inport  Port=4
  Gate In Ext : Inport  Port=5
  Convert : xbsIndex_r4/Convert  arith_type=Boolean  n_bits=16  bin_pt=14  quantization=Truncate  overflow=Wrap  latency=0  dbl_ovrd=off  pipeline=off  block_type=convert
      settings: block_version=8.2
  Counter : xbsIndex_r4/Counter  cnt_type=Free Running  cnt_to=Inf  operation=Up  start_count=0  cnt_by_val=1  arith_type=Unsigned  n_bits=1  bin_pt=0  load_pin=off  rst=on  en=on  explicit_period=on  period=1/60e6  dbl_ovrd=off  use_behavioral_HDL=off  use_rpm=off  block_type=counter
      settings: block_version=8.2
  Delay : xbsIndex_r4/Delay  en=off  latency=1  dbl_ovrd=off  reg_retiming=off  block_type=delay
      settings: infoedit=Hardware notes: A delay line is a chain, each link of which is an SRL16 followed by a flip-flop. If register retiming is enabled, the delay line is a chain of flip-flops.  block_version=8.2
  Delay1 : xbsIndex_r4/Delay  en=off  latency=279  dbl_ovrd=off  reg_retiming=off  block_type=delay
      settings: infoedit=Hardware notes: A delay line is a chain, each link of which is an SRL16 followed by a flip-flop. If register retiming is enabled, the delay line is a chain of flip-flops.  block_version=8.2
  Delay2 : xbsIndex_r4/Delay  en=off  latency=279  dbl_ovrd=off  reg_retiming=off  block_type=delay
      settings: infoedit=Hardware notes: A delay line is a chain, each link of which is an SRL16 followed by a flip-flop. If register retiming is enabled, the delay line is a chain of flip-flops.  block_version=8.2
  Delay3 : xbsIndex_r4/Delay  en=off  latency=1  dbl_ovrd=off  reg_retiming=off  block_type=delay
      settings: infoedit=Hardware notes: A delay line is a chain, each link of which is an SRL16 followed by a flip-flop. If register retiming is enabled, the delay line is a chain of flip-flops.  block_version=8.2
  Delay4 : xbsIndex_r4/Delay  en=off  latency=1  dbl_ovrd=off  reg_retiming=off  block_type=delay
      settings: infoedit=Hardware notes: A delay line is a chain, each link of which is an SRL16 followed by a flip-flop. If register retiming is enabled, the delay line is a chain of flip-flops.  block_version=8.2
  Inverter : xbsIndex_r4/Inverter  en=off  latency=0  dbl_ovrd=off  block_type=inv
      settings: block_version=8.2
  Logical : xbsIndex_r4/Logical  logical_function=OR  inputs=2  en=off  latency=0  precision=Full  arith_type=Unsigned  n_bits=16  bin_pt=0  align_bp=on  dbl_ovrd=off  block_type=logical
      settings: block_version=8.2
  Logical1 : xbsIndex_r4/Logical  logical_function=XOR  inputs=2  en=off  latency=0  precision=Full  arith_type=Unsigned  n_bits=16  bin_pt=0  align_bp=on  dbl_ovrd=off  block_type=logical
      settings: block_version=8.2
  Logical2 : xbsIndex_r4/Logical  logical_function=AND  inputs=2  en=off  latency=0  precision=Full  arith_type=Unsigned  n_bits=16  bin_pt=0  align_bp=on  dbl_ovrd=off  block_type=logical
      settings: block_version=8.2
  Logical3 : xbsIndex_r4/Logical  logical_function=AND  inputs=2  en=off  latency=0  precision=Full  arith_type=Unsigned  n_bits=16  bin_pt=0  align_bp=on  dbl_ovrd=off  block_type=logical
      settings: block_version=8.2
  Logical4 : xbsIndex_r4/Logical  logical_function=AND  inputs=2  en=off  latency=0  precision=Full  arith_type=Unsigned  n_bits=16  bin_pt=0  align_bp=on  dbl_ovrd=off  block_type=logical
      settings: block_version=8.2
  Mux : xbsIndex_r4/Mux  inputs=2  en=off  latency=0  precision=Full  arith_type=Unsigned  n_bits=16  bin_pt=14  quantization=Truncate  overflow=Wrap  dbl_ovrd=off  block_type=mux
      settings: block_version=8.2
  Gate 1 Out : Outport
  Gate 2 Out : Outport  Port=2
  wires:
  Timing Sel/1 -> Mux/1
  Gate In Ext/1 -> Delay3/1
  Gate In Int/1 -> Delay4/1
  Mux/1 -> Delay/1, Logical/2, Logical2/2, Logical1/2, Logical3/2
  Delay/1 -> Logical/1
  Logical/1 -> Logical1/1
  Counter/1 -> Convert/1
  Inverter/1 -> Logical2/1
  Logical3/1 -> Delay2/1
  Logical2/1 -> Delay1/1
  Convert/1 -> Inverter/1, Logical3/1
  Logical1/1 -> Logical4/2
  Dual PRT/1 -> Logical4/1
  Logical4/1 -> Counter/2
  Reset/1 -> Counter/1
  Delay1/1 -> Gate 1 Out/1
  Delay2/1 -> Gate 2 Out/1
  Delay3/1 -> Mux/2
  Delay4/1 -> Mux/3

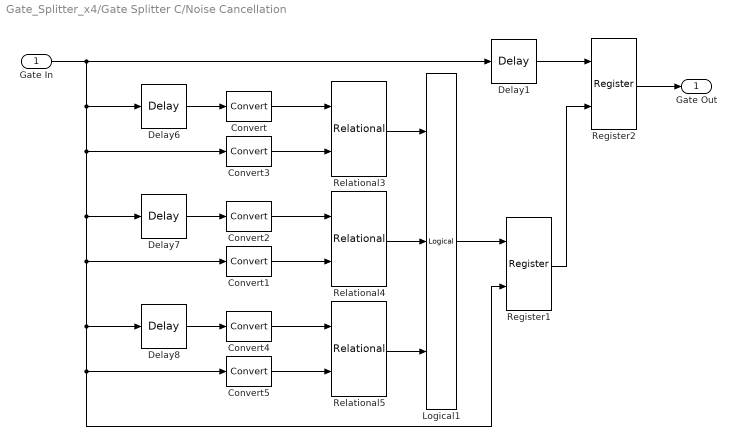
== system Gate_Splitter_x4/Gate Splitter C/Noise Cancellation ==
  Gate In : Inport
  Convert{,1..5} (6 alike) : xbsIndex_r4/Convert  arith_type=Unsigned  n_bits=1  bin_pt=0  quantization=Truncate  overflow=Saturate  latency=0  dbl_ovrd=off  pipeline=off  block_type=convert
      settings: block_version=8.2
  Delay1 : xbsIndex_r4/Delay  en=off  latency=4  dbl_ovrd=off  reg_retiming=off  block_type=delay
      settings: infoedit=Hardware notes: A delay line is a chain, each link of which is an SRL16 followed by a flip-flop. If register retiming is enabled, the delay line is a chain of flip-flops.  block_version=8.2
  Delay6 : xbsIndex_r4/Delay  en=off  latency=1  dbl_ovrd=off  reg_retiming=off  block_type=delay
      settings: infoedit=Hardware notes: A delay line is a chain, each link of which is an SRL16 followed by a flip-flop. If register retiming is enabled, the delay line is a chain of flip-flops.  block_version=8.2
  Delay7 : xbsIndex_r4/Delay  en=off  latency=2  dbl_ovrd=off  reg_retiming=off  block_type=delay
      settings: infoedit=Hardware notes: A delay line is a chain, each link of which is an SRL16 followed by a flip-flop. If register retiming is enabled, the delay line is a chain of flip-flops.  block_version=8.2
  Delay8 : xbsIndex_r4/Delay  en=off  latency=3  dbl_ovrd=off  reg_retiming=off  block_type=delay
      settings: infoedit=Hardware notes: A delay line is a chain, each link of which is an SRL16 followed by a flip-flop. If register retiming is enabled, the delay line is a chain of flip-flops.  block_version=8.2
  Logical1 : xbsIndex_r4/Logical  logical_function=OR  inputs=3  en=off  latency=0  precision=Full  arith_type=Unsigned  n_bits=16  bin_pt=0  align_bp=on  dbl_ovrd=off  block_type=logical
      settings: block_version=8.2
  Register1 : xbsIndex_r4/Register  init=0  rst=off  en=on  dbl_ovrd=off  block_type=register
      settings: block_version=8.2
  Register2 : xbsIndex_r4/Register  init=0  rst=on  en=off  dbl_ovrd=off  block_type=register
      settings: block_version=8.2
  Relational3 : xbsIndex_r4/Relational  mode=a!=b  en=off  latency=2  dbl_ovrd=off  block_type=relational
      settings: block_version=8.2
  Relational4 : xbsIndex_r4/Relational  mode=a!=b  en=off  latency=1  dbl_ovrd=off  block_type=relational
      settings: block_version=8.2
  Relational5 : xbsIndex_r4/Relational  mode=a!=b  en=off  latency=0  dbl_ovrd=off  block_type=relational
      settings: block_version=8.2
  Gate Out : Outport
  wires:
  Convert/1 -> Relational3/1
  Delay6/1 -> Convert/1
  Convert2/1 -> Relational4/1
  Delay7/1 -> Convert2/1
  Convert4/1 -> Relational5/1
  Delay8/1 -> Convert4/1
  Convert5/1 -> Relational5/2
  Relational3/1 -> Logical1/1
  Relational4/1 -> Logical1/2
  Relational5/1 -> Logical1/3
  Convert3/1 -> Relational3/2
  Convert1/1 -> Relational4/2
  Delay1/1 -> Register2/1
  Logical1/1 -> Register1/1
  Register1/1 -> Register2/2
  Gate In/1 -> Delay6/1, Delay7/1, Delay8/1, Convert5/1, Register1/2, Convert1/1, Convert3/1, Delay1/1
  Register2/1 -> Gate Out/1

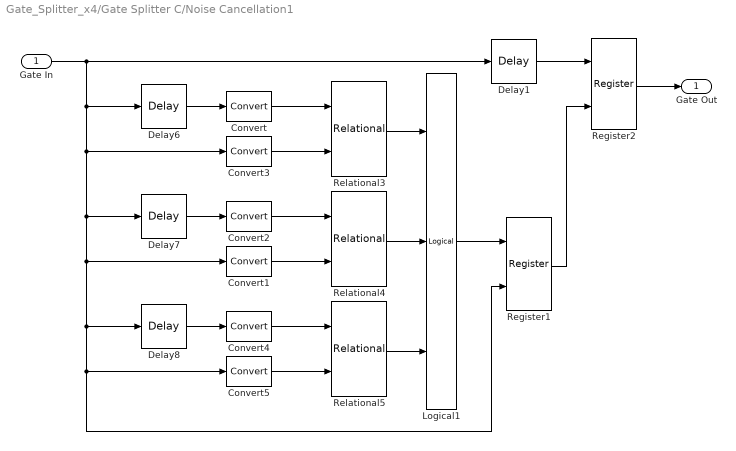
== system Gate_Splitter_x4/Gate Splitter C/Noise Cancellation1 ==
  Gate In : Inport
  Convert{,1..5} (6 alike) : xbsIndex_r4/Convert  arith_type=Unsigned  n_bits=1  bin_pt=0  quantization=Truncate  overflow=Saturate  latency=0  dbl_ovrd=off  pipeline=off  block_type=convert
      settings: block_version=8.2
  Delay1 : xbsIndex_r4/Delay  en=off  latency=4  dbl_ovrd=off  reg_retiming=off  block_type=delay
      settings: infoedit=Hardware notes: A delay line is a chain, each link of which is an SRL16 followed by a flip-flop. If register retiming is enabled, the delay line is a chain of flip-flops.  block_version=8.2
  Delay6 : xbsIndex_r4/Delay  en=off  latency=1  dbl_ovrd=off  reg_retiming=off  block_type=delay
      settings: infoedit=Hardware notes: A delay line is a chain, each link of which is an SRL16 followed by a flip-flop. If register retiming is enabled, the delay line is a chain of flip-flops.  block_version=8.2
  Delay7 : xbsIndex_r4/Delay  en=off  latency=2  dbl_ovrd=off  reg_retiming=off  block_type=delay
      settings: infoedit=Hardware notes: A delay line is a chain, each link of which is an SRL16 followed by a flip-flop. If register retiming is enabled, the delay line is a chain of flip-flops.  block_version=8.2
  Delay8 : xbsIndex_r4/Delay  en=off  latency=3  dbl_ovrd=off  reg_retiming=off  block_type=delay
      settings: infoedit=Hardware notes: A delay line is a chain, each link of which is an SRL16 followed by a flip-flop. If register retiming is enabled, the delay line is a chain of flip-flops.  block_version=8.2
  Logical1 : xbsIndex_r4/Logical  logical_function=OR  inputs=3  en=off  latency=0  precision=Full  arith_type=Unsigned  n_bits=16  bin_pt=0  align_bp=on  dbl_ovrd=off  block_type=logical
      settings: block_version=8.2
  Register1 : xbsIndex_r4/Register  init=0  rst=off  en=on  dbl_ovrd=off  block_type=register
      settings: block_version=8.2
  Register2 : xbsIndex_r4/Register  init=0  rst=on  en=off  dbl_ovrd=off  block_type=register
      settings: block_version=8.2
  Relational3 : xbsIndex_r4/Relational  mode=a!=b  en=off  latency=2  dbl_ovrd=off  block_type=relational
      settings: block_version=8.2
  Relational4 : xbsIndex_r4/Relational  mode=a!=b  en=off  latency=1  dbl_ovrd=off  block_type=relational
      settings: block_version=8.2
  Relational5 : xbsIndex_r4/Relational  mode=a!=b  en=off  latency=0  dbl_ovrd=off  block_type=relational
      settings: block_version=8.2
  Gate Out : Outport
  wires:
  Convert/1 -> Relational3/1
  Delay6/1 -> Convert/1
  Convert2/1 -> Relational4/1
  Delay7/1 -> Convert2/1
  Convert4/1 -> Relational5/1
  Delay8/1 -> Convert4/1
  Convert5/1 -> Relational5/2
  Relational3/1 -> Logical1/1
  Relational4/1 -> Logical1/2
  Relational5/1 -> Logical1/3
  Convert3/1 -> Relational3/2
  Convert1/1 -> Relational4/2
  Delay1/1 -> Register2/1
  Logical1/1 -> Register1/1
  Register1/1 -> Register2/2
  Gate In/1 -> Delay6/1, Delay7/1, Delay8/1, Convert5/1, Register1/2, Convert1/1, Convert3/1, Delay1/1
  Register2/1 -> Gate Out/1
